simulink model "SlidControlSatSim"  (R2018a)
settings: Solver=VariableStepAuto  StartTime=0.0  StopTime=20  RelTol=1e-3
values from neighbouring files (symbols this model uses):
  A = [a 0;1 0]    [SlidingControl.m]
  B = [b;0]    [SlidingControl.m]
  D = [1;0]    [SlidingControl.m]
  dmax = 0.9    [SlidingControl.m]
  Mu = 0.5    [SlidingControl.m]
  surf_C = [c1;c2]    [SlidingControl.m]
settings Model: Creator=ageng  LastModifiedBy=ageng

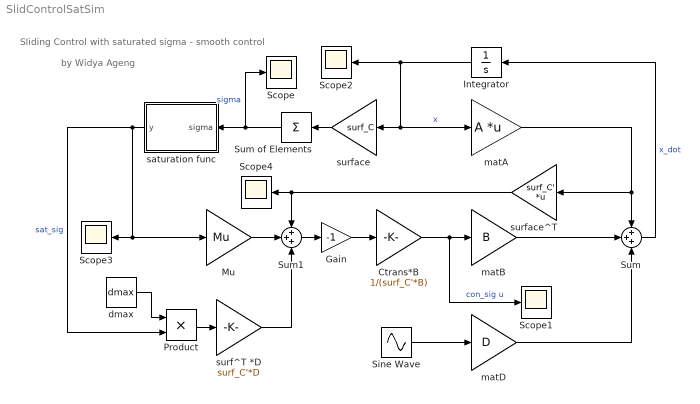
== system SlidControlSatSim ==
  note: by Widya Ageng
  note: Sliding Control with saturated sigma - smooth control
  "Ctrans*B " : Gain  Gain=1/(surf_C'*B)
  Gain : Gain  Gain=-1
  Integrator : Integrator  InitialCondition=[1.5;1.5]
  Mu : Gain  Gain=Mu
  Product : Product
  Scope{,1..4} (5 alike) : Scope
  Sine Wave : Sin  Amplitude=dmax  Frequency=628  SampleTime=0
  Sum : Sum  Inputs=+++
  Sum of Elements : Sum  Inputs=+
  Sum1 : Sum  Inputs=+++
  dmax : Constant  Value=dmax  SampleTime=0.0001
  matA : Gain  Gain=A  Multiplication=Matrix(K*u) (u vector)
  matB : Gain  Gain=B
  matD : Gain  Gain=D
  saturation func : MATLAB Function  TreatAsAtomicUnit=on
  surf^T *D : Gain  Gain=surf_C'*D
  "surface " : Gain  Gain=surf_C
  surface^T : Gain  Gain=surf_C'  Multiplication=Matrix(K*u) (u vector)
  wires:
  Integrator/1 -> Scope2/1, "surface "/1, matA/1  "x"
  matA/1 -> surface^T/1, Sum/1
  matB/1 -> Sum/2
  matD/1 -> Sum/3
  Sum/1 -> Integrator/1  "x_dot"
  surface^T/1 -> Scope4/1, Sum1/1
  Sum of Elements/1 -> saturation func/1(sigma), Scope/1  "sigma"
  "surface "/1 -> Sum of Elements/1
  Mu/1 -> Sum1/2
  saturation func/1(y) -> Mu/1, Scope3/1, Product/2  "sat_sig"
  Sum1/1 -> Gain/1
  Gain/1 -> "Ctrans*B "/1
  "Ctrans*B "/1 -> Scope1/1, matB/1  "con_sig u"
  Sine Wave/1 -> matD/1
  surf^T *D/1 -> Sum1/3
  Product/1 -> surf^T *D/1
  dmax/1 -> Product/1

== matlab function SlidControlSatSim/saturation func ==
  data: sigma input; y output
function y = fcn(sigma)

epsilon = 0.01;

if sigma>epsilon
    out = 1;
elseif sigma<(-1)*epsilon
    out = -1;
else
    out = sigma/epsilon;
end

y = out;
